simulink model "HW01_revised02_model_2023_1114_PI"  (R2023b)
settings: Solver=VariableStepAuto  StartTime=0.0  StopTime=50  RelTol=1e-3
libraries: slpidlib x1
settings Model: Creator=admin  LastModifiedBy=YYlab_05

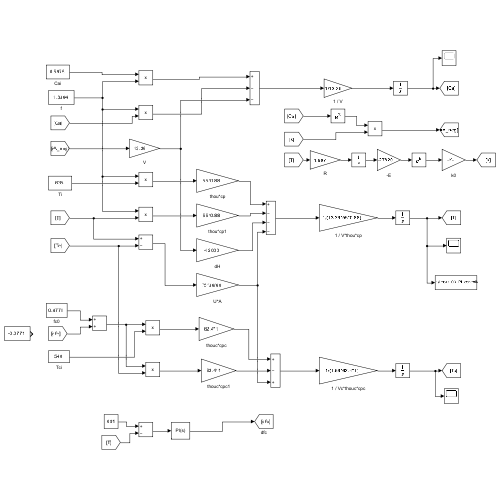
[thumbnail: Simulink's stored preview of the top-level diagram]
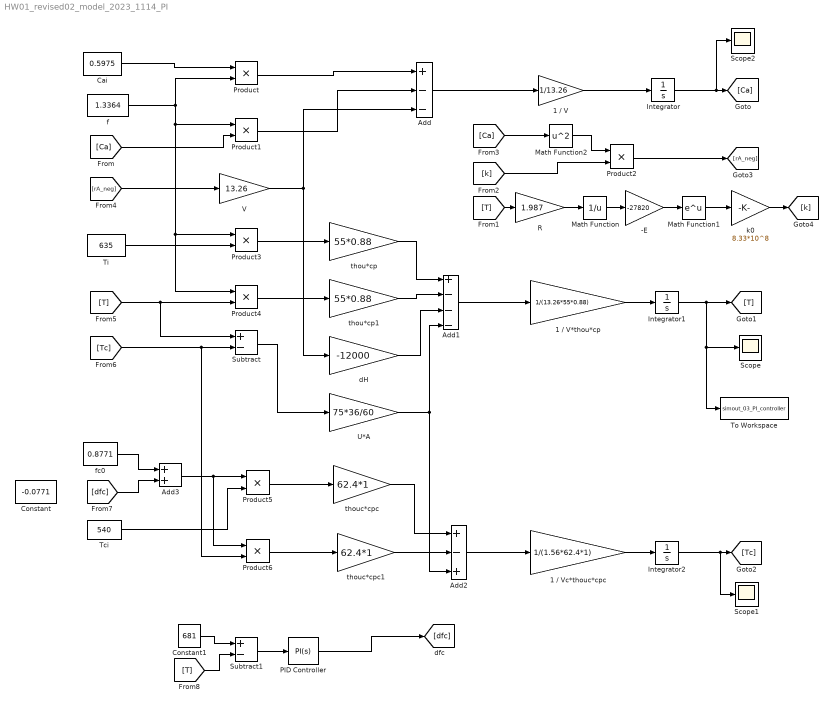
== system HW01_revised02_model_2023_1114_PI ==
  -E : Gain  Gain=-27820
  1 / V : Gain  Gain=1/13.26
  1 / V*thou*cp : Gain  Gain=1/(13.26*55*0.88)
  1 / Vc*thouc*cpc : Gain  Gain=1/(1.56*62.4*1)
  Add : Sum  Inputs=+--
  Add1 : Sum  Inputs=+---
  Add2 : Sum  Inputs=+-+
  Add3 : Sum
  Cai : Constant  Value=0.5975
  Constant : Constant  Value=-0.0771
  Constant1 : Constant  Value=681
  Integrator : Integrator  InitialCondition=0.2068
  Integrator1 : Integrator  InitialCondition=678.9
  Integrator2 : Integrator  InitialCondition=602.7
  Math Function : Math  Operator=reciprocal
  Math Function1 : Math
  Math Function2 : Math  Operator=square
  PID Controller : slpidlib/PID Controller  Controller=PI  Form=Parallel  TimeDomain=Continuous-time  UseExternalTs=off  SampleTime=-1  IntegratorMethod=Forward Euler  FilterMethod=Forward Euler  ControllerParametersSource=internal  P=-0.4174  I=-0.2087  UseKiTs=off  D=0  N=100  UseFilter=on  TunerSelectOption=Transfer Function Based (PID Tuner App)  InitialConditionSource=internal  InitialConditionForIntegrator=0  InitialConditionForFilter=0  DifferentiatorICPrevScaledInput=0  ExternalReset=none  TrackingMode=off  Kt=1  LimitOutput=off  SatLimitsSource=internal  UpperSaturationLimit=inf  LowerSaturationLimit=-inf  LinearizeAsGain=on  AntiWindupMode=none  Kb=1  LimitIntegrator=off  UpperIntegratorSaturationLimit=inf  LowerIntegratorSaturationLimit=-inf  POutMin=[]  POutMax=[]  IOutMin=[]  IOutMax=[]  DOutMin=[]  DOutMax=[]  NOutMin=[]  NOutMax=[]  SumOutMin=[]  SumOutMax=[]  SaturationOutMin=[]  SaturationOutMax=[]  PParamMin=[]  PParamMax=[]  IParamMin=[]  IParamMax=[]  DParamMin=[]  DParamMax=[]  NParamMin=[]  NParamMax=[]  KbParamMin=[]  KbParamMax=[]  KtParamMin=[]  KtParamMax=[]  KbOutMin=[]  KbOutMax=[]  KtOutMin=[]  KtOutMax=[]  IntegratorOutMin=[]  IntegratorOutMax=[]  FilterOutMin=[]  FilterOutMax=[]  SumI1OutMin=[]  SumI1OutMax=[]  SumI2OutMin=[]  SumI2OutMax=[]  SumI3OutMin=[]  SumI3OutMax=[]  SumI4OutMin=[]  SumI4OutMax=[]  SumDOutMin=[]  SumDOutMax=[]  DifferentiatorOutMin=[]  DifferentiatorOutMax=[]  FilterDiffOutCoefMin=[]  FilterDiffOutCoefMax=[]  ReciprocalOutMin=[]  ReciprocalOutMax=[]  SumDenOutMin=[]  SumDenOutMax=[]  SumNumOutMin=[]  SumNumOutMax=[]  DivideOutMin=[]  DivideOutMax=[]  UdiffTsProdOutMin=[]  UdiffTsProdOutMax=[]  NTsProdOutMin=[]  NTsProdOutMax=[]  UintegralTsProdOutMin=[]  UintegralTsProdOutMax=[]  UngainTsProdOutMin=[]  UngainTsProdOutMax=[]  ClampingZeroOutDataTypeStr=Inherit: Inherit via back propagation  ClampingZeroOutMin=[]  ClampingZeroOutMax=[]  FilterDenConstantOutDataTypeStr=Inherit: Inherit via back propagation  FilterDenConstantOutMin=[]  FilterDenConstantOutMax=[]  PCopyOutDataTypeStr=Inherit: Inherit via back propagation  PCopyOutMin=[]  PCopyOutMax=[]  NCopyOutDataTypeStr=Inherit: Inherit via back propagation  NCopyOutMin=[]  NCopyOutMax=[]  IntegratorContinuousStateAttributes=''  IntegratorStateMustResolveToSignalObject=off  IntegratorRTWStateStorageClass=Auto  FilterContinuousStateAttributes=''  FilterStateMustResolveToSignalObject=off  FilterRTWStateStorageClass=Auto  ParallelPVariant=InternalParameters  IdealPVariant=Disabled  IVariant=InternalParameters  DVariant=Disabled  IntegratorVariant=Continuous  SatVariant=Disabled  AWVariant=Passthrough  PCopyVariant=Disabled  TRVariant=Disabled  FdbkBlocksVariant=Forward  IdealPFdbkVariant=Disabled  SatFdbkVariant=Disabled  DerivativeFilterVariant=Disabled  NVariant=Disabled  NCopyVariant=Disabled_SignalSpec  FilterICVariant=Disabled  IntegratorICVariant=InternalICs  ExternalResetVariant=Disabled  TRSumVariant=Passthrough  SumFdbkVariant=Disabled  SumVariant=Sum_PI  TsampFilterVariant=InternalTs  TsampNgainVariant=Passthrough  TsampIntegralVariant=Disabled_SignalSpec  ExternalSaturationOutDataTypeStr=Inherit: Same as second input
  Product{,1..6} (7 alike) : Product
  "R " : Gain  Gain=1.987
  Scope : Scope
  Scope1 : Scope
  Scope2 : Scope
  Subtract : Sum  Inputs=+-
  Subtract1 : Sum  Inputs=+-
  Tci : Constant  Value=540
  Ti : Constant  Value=635
  To Workspace : ToWorkspace  VariableName=simout_03_PI_controller  SaveFormat=Timeseries  SampleTime=-1
  U*A : Gain  Gain=75*36/60
  V : Gain  Gain=13.26
  dH : Gain  Gain=-12000
  f : Constant  Value=1.3364
  fc0 : Constant  Value=0.8771
  k0 : Gain  Gain=8.33*10^8
  thou*cp : Gain  Gain=55*0.88
  thou*cp1 : Gain  Gain=55*0.88
  thouc*cpc : Gain  Gain=62.4*1
  thouc*cpc1 : Gain  Gain=62.4*1
  wires:
  Integrator/1 -> Scope2/1, [Ca]
  Integrator1/1 -> To Workspace/1, Scope/1, [T]
  Integrator2/1 -> Scope1/1, [Tc]
  1 / V/1 -> Integrator/1
  Cai/1 -> Product/1
  f/1 -> Product1/1, Product4/1, Product3/1, Product/2
  Product/1 -> Add/1
  [Ca] -> Product1/2
  Product1/1 -> Add/2
  [T] -> "R "/1
  "R "/1 -> Math Function/1
  Math Function/1 -> -E/1
  -E/1 -> Math Function1/1
  Math Function1/1 -> k0/1
  [Ca] -> Math Function2/1
  Math Function2/1 -> Product2/1
  [k] -> Product2/2
  Product2/1 -> [rA_neg]
  [rA_neg] -> V/1
  V/1 -> dH/1, Add/3
  Add/1 -> 1 / V/1
  1 / V*thou*cp/1 -> Integrator1/1
  Ti/1 -> Product3/2
  Product3/1 -> thou*cp/1
  thou*cp/1 -> Add1/1
  [T] -> Subtract/1, Product4/2
  Product4/1 -> thou*cp1/1
  thou*cp1/1 -> Add1/2
  Add1/1 -> 1 / V*thou*cp/1
  dH/1 -> Add1/3
  U*A/1 -> Add1/4, Add2/3
  [Tc] -> Product6/2, Subtract/2
  Subtract/1 -> U*A/1
  Add2/1 -> 1 / Vc*thouc*cpc/1
  1 / Vc*thouc*cpc/1 -> Integrator2/1
  fc0/1 -> Add3/1
  [dfc] -> Add3/2
  Add3/1 -> Product6/1, Product5/1
  Tci/1 -> Product5/2
  Product5/1 -> thouc*cpc/1
  thouc*cpc/1 -> Add2/1
  Product6/1 -> thouc*cpc1/1
  thouc*cpc1/1 -> Add2/2
  k0/1 -> [k]
  Constant1/1 -> Subtract1/1
  [T] -> Subtract1/2
  Subtract1/1 -> PID Controller/1
  PID Controller/1 -> [dfc]
